simulink model "control_pra"  (R2021a)
settings: Solver=FixedStepDiscrete  StartTime=0.0  StopTime=10  FixedStep=0.005  RelTol=1e-3  EnableMultiTasking=on
PreLoadFcn:
  | disp(pwd)
PostLoadFcn:
  | c2000demoscallback(1)
undefined symbols (not defined in the file): CommandConstEnable, CommandData, FrameData, MailBoxRx, MailBoxTx, SCIAReceivedComplete, StatusConstClose, StatusConstClosed, StatusConstError, StatusConstHoming, StatusConstIdle, StatusConstPaused, StatusConstReady, StatusConstReset, StatusConstRunning, StatusConstStart, StatusConstStopped, StatusData
libraries: simulink x30, c280xlib x19, idelinklib_common x16, c2000lib x1, c2833xlib x1
(part 3 of 3)

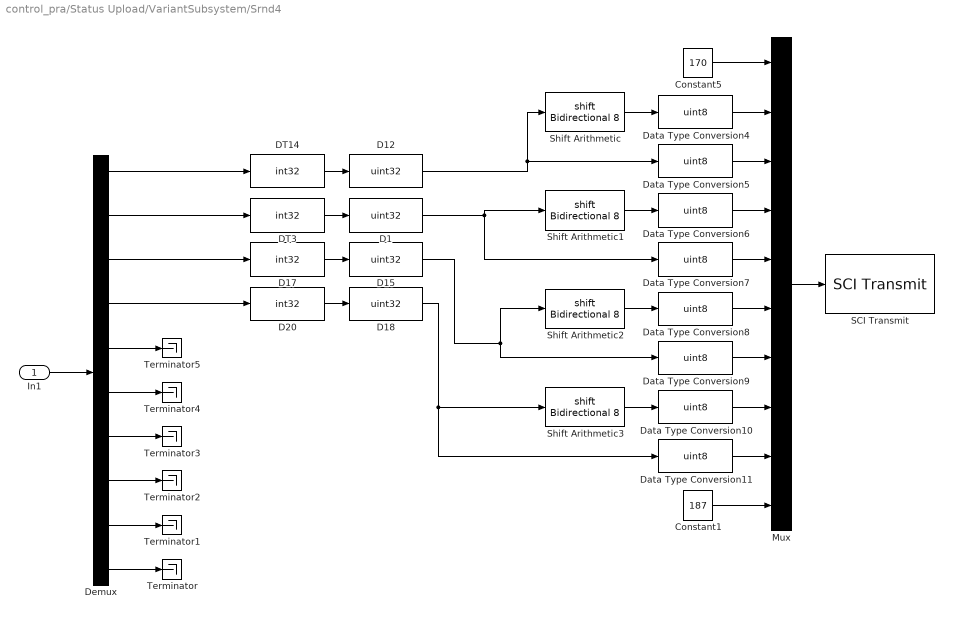
== system control_pra/Status Upload/VariantSubsystem/Srnd4 ==
  In1 : Inport
  Constant1 : Constant  Value=187  OutDataTypeStr=uint8
  Constant5 : Constant  Value=170  OutDataTypeStr=uint8
  D{1,12,15,18} (4 alike) : DataTypeConversion  OutDataTypeStr=uint32
  D17 : DataTypeConversion  OutDataTypeStr=int32
  D20 : DataTypeConversion  OutDataTypeStr=int32
  DT14 : DataTypeConversion  OutDataTypeStr=int32
  DT3 : DataTypeConversion  OutDataTypeStr=int32
  Data Type Conversion{4..11} (8 alike) : DataTypeConversion  OutDataTypeStr=uint8
  Demux : Demux  Outputs=10
  Mux : Mux  Inputs=10
  SCI Transmit : c280xlib/SCI Transmit  sciModule=A  dataHead=''  dataTail=''  postInterrupt=on  numFifo=16
  Shift Arithmetic{,1..3} (4 alike) : ArithShift  BitShiftNumber=8
  Terminator{,1..5} (6 alike) : Terminator
  wires:
  In1/1 -> Demux/1
  Demux/3 -> D17/1
  Demux/1 -> DT14/1
  Demux/2 -> DT3/1
  Demux/4 -> D20/1
  Demux/10 -> Terminator/1
  Demux/9 -> Terminator1/1
  Demux/8 -> Terminator2/1
  Demux/7 -> Terminator3/1
  Demux/6 -> Terminator4/1
  Demux/5 -> Terminator5/1
  DT14/1 -> D12/1
  DT3/1 -> D1/1
  D17/1 -> D15/1
  D20/1 -> D18/1
  Data Type Conversion11/1 -> Mux/9
  Data Type Conversion9/1 -> Mux/7
  Shift Arithmetic2/1 -> Data Type Conversion8/1
  Data Type Conversion7/1 -> Mux/5
  D18/1 -> Data Type Conversion11/1, Shift Arithmetic3/1
  D1/1 -> Data Type Conversion7/1, Shift Arithmetic1/1
  Shift Arithmetic/1 -> Data Type Conversion4/1
  Data Type Conversion8/1 -> Mux/6
  Constant1/1 -> Mux/10
  Data Type Conversion4/1 -> Mux/2
  Shift Arithmetic3/1 -> Data Type Conversion10/1
  Data Type Conversion6/1 -> Mux/4
  Constant5/1 -> Mux/1
  Mux/1 -> SCI Transmit/1
  D15/1 -> Data Type Conversion9/1, Shift Arithmetic2/1
  D12/1 -> Shift Arithmetic/1, Data Type Conversion5/1
  Data Type Conversion5/1 -> Mux/3
  Data Type Conversion10/1 -> Mux/8
  Shift Arithmetic1/1 -> Data Type Conversion6/1

== system control_pra/System Config/CAN_Config_C/Model Header ==

== system control_pra/System Config/CAN_Config_C/Model Source1 ==

== system control_pra/System Config/CAN_Config_C/System Initialize1 ==

== system control_pra/System Config/CAN_Config_S/Model Header ==

== system control_pra/System Config/CAN_Config_S/Model Source1 ==

== system control_pra/System Config/CAN_Config_S/Subsystem ==
  Enable : EnablePort
  eCANAM0 : c280xlib/eCAN Transmit  chipFamily=C280x  useModule=eCAN_A  mailboxNo=0  messageID=hex2dec('300')  messageType=Standard (11-bit identifier)  enableBlockingMode=off  postInterrupt=off  interruptLine=0
      settings: SourceProductBaseCode=TIC2000
  eCANAM1 : c280xlib/eCAN Transmit  chipFamily=C280x  useModule=eCAN_A  mailboxNo=1  messageID=hex2dec('301')  messageType=Standard (11-bit identifier)  enableBlockingMode=off  postInterrupt=off  interruptLine=0
      settings: SourceProductBaseCode=TIC2000
  eCANAM2 : c280xlib/eCAN Transmit  Commented=on  chipFamily=C280x  useModule=eCAN_A  mailboxNo=2  messageID=hex2dec('301')  messageType=Standard (11-bit identifier)  enableBlockingMode=off  postInterrupt=off  interruptLine=0
      settings: SourceProductBaseCode=TIC2000
  eCANAM3 : c280xlib/eCAN Transmit  Commented=on  chipFamily=C280x  useModule=eCAN_A  mailboxNo=3  messageID=hex2dec('303')  messageType=Standard (11-bit identifier)  enableBlockingMode=off  postInterrupt=off  interruptLine=0
      settings: SourceProductBaseCode=TIC2000
  eCANAM4 : c280xlib/eCAN Receive  chipFamily=C280x  useModule=eCAN_A  mailboxNo=4  messageID=hex2dec('281')  messageType=Standard (11-bit identifier)  sampleTime=-1  dataType=uint16  initValue=0  outputMessageLength=off  outputMessageTimeStamp=off  postInterrupt=off  interruptLine=0
      settings: SourceProductBaseCode=TIC2000
  eCANAM5 : c280xlib/eCAN Receive  Commented=on  chipFamily=C280x  useModule=eCAN_A  mailboxNo=5  messageID=hex2dec('281')  messageType=Standard (11-bit identifier)  sampleTime=-1  dataType=uint16  initValue=0  outputMessageLength=off  outputMessageTimeStamp=off  postInterrupt=off  interruptLine=0
      settings: SourceProductBaseCode=TIC2000
  eCANAM6 : c280xlib/eCAN Receive  Commented=on  chipFamily=C280x  useModule=eCAN_A  mailboxNo=6  messageID=hex2dec('283')  messageType=Standard (11-bit identifier)  sampleTime=-1  dataType=uint16  initValue=0  outputMessageLength=off  outputMessageTimeStamp=off  postInterrupt=off  interruptLine=0
      settings: SourceProductBaseCode=TIC2000
  eCANBM0 : c280xlib/eCAN Transmit  Commented=on  chipFamily=C280x  useModule=eCAN_B  mailboxNo=0  messageID=hex2dec('300')  messageType=Standard (11-bit identifier)  enableBlockingMode=off  postInterrupt=off  interruptLine=0
      settings: SourceProductBaseCode=TIC2000
  eCANBM1 : c280xlib/eCAN Transmit  Commented=on  chipFamily=C280x  useModule=eCAN_B  mailboxNo=1  messageID=hex2dec('304')  messageType=Standard (11-bit identifier)  enableBlockingMode=off  postInterrupt=off  interruptLine=0
      settings: SourceProductBaseCode=TIC2000
  eCANBM2 : c280xlib/eCAN Transmit  Commented=on  chipFamily=C280x  useModule=eCAN_B  mailboxNo=2  messageID=hex2dec('305')  messageType=Standard (11-bit identifier)  enableBlockingMode=off  postInterrupt=off  interruptLine=0
      settings: SourceProductBaseCode=TIC2000
  eCANBM3 : c280xlib/eCAN Transmit  Commented=on  chipFamily=C280x  useModule=eCAN_B  mailboxNo=3  messageID=hex2dec('306')  messageType=Standard (11-bit identifier)  enableBlockingMode=off  postInterrupt=off  interruptLine=0
      settings: SourceProductBaseCode=TIC2000
  eCANBM4 : c280xlib/eCAN Receive  Commented=on  chipFamily=C280x  useModule=eCAN_B  mailboxNo=4  messageID=hex2dec('284')  messageType=Standard (11-bit identifier)  sampleTime=-1  dataType=uint16  initValue=0  outputMessageLength=off  outputMessageTimeStamp=off  postInterrupt=off  interruptLine=0
      settings: SourceProductBaseCode=TIC2000
  eCANBM5 : c280xlib/eCAN Receive  Commented=on  chipFamily=C280x  useModule=eCAN_B  mailboxNo=5  messageID=hex2dec('285')  messageType=Standard (11-bit identifier)  sampleTime=-1  dataType=uint16  initValue=0  outputMessageLength=off  outputMessageTimeStamp=off  postInterrupt=off  interruptLine=0
      settings: SourceProductBaseCode=TIC2000
  eCANBM6 : c280xlib/eCAN Receive  Commented=on  chipFamily=C280x  useModule=eCAN_B  mailboxNo=6  messageID=hex2dec('286')  messageType=Standard (11-bit identifier)  sampleTime=-1  dataType=uint16  initValue=0  outputMessageLength=off  outputMessageTimeStamp=off  postInterrupt=off  interruptLine=0
      settings: SourceProductBaseCode=TIC2000

== system control_pra/System Config/CAN_Config_S/System Initialize1 ==

== system control_pra/System Config/CAN_Config_S/eCANA Transmit1 ==
  Data : Inport
  Constant1 : Constant  Value=MailBox  OutDataTypeStr=uint8  SampleTime=-1
  Memory Copy : idelinklib_common/Memory Copy  copyFrom=Input port  copyFromAddressSource=Specify via dialog  copyFromAddress=hex2dec('00001000')  copyFromSrcCode=myVariableSrc  dataTypeFrom=Inherit from input port  dataDimensionFrom=4  useOffsetFrom=off  offsetFromSrc=Specify via dialog  offsetFrom=0  strideFrom=1  copyTo=Specified source code symbol  copyToAddressSource=Specify via dialog  copyToAddress=hex2dec('00002000')  copyToSrcCode=&CanAMsg.TxWord  dataTypeTo=uint16  useOffsetTo=off  offsetToSrc=Specify via dialog  offsetTo=0  strideTo=1  sampleTime=-1  useInitValue=off  initValueSrc=Specify constant value  initValue=1  initValueSrcCode=myInitValueVariable  useAsMask=off  maskOperator=bitwise AND  useTermValue=off  termValue=1  isRealtimeEnabled=off  emitCCBeforeWrite=off  CCBeforeWrite=/* Custom Code Before Write*/  emitCCAfterWrite=off  CCAfterWrite=/* Custom Code After Write*/  useDMACopy=off  enableBlockingMode=off
      settings: SourceProductBaseCode=ME
  Memory Copy1 : idelinklib_common/Memory Copy  copyFrom=Input port  copyFromAddressSource=Specify via dialog  copyFromAddress=hex2dec('00001000')  copyFromSrcCode=myVariableSrc  dataTypeFrom=Inherit from input port  dataDimensionFrom=1  useOffsetFrom=off  offsetFromSrc=Specify via dialog  offsetFrom=0  strideFrom=1  copyTo=Specified source code symbol  copyToAddressSource=Specify via dialog  copyToAddress=hex2dec('00002000')  copyToSrcCode=&CanAMsg.MailBox  dataTypeTo=uint8  useOffsetTo=off  offsetToSrc=Specify via dialog  offsetTo=0  strideTo=1  sampleTime=-1  useInitValue=off  initValueSrc=Specify constant value  initValue=1  initValueSrcCode=myInitValueVariable  useAsMask=off  maskOperator=bitwise AND  useTermValue=off  termValue=1  isRealtimeEnabled=off  emitCCBeforeWrite=off  CCBeforeWrite=/* Custom Code Before Write*/  emitCCAfterWrite=off  CCAfterWrite=/* Custom Code After Write*/  useDMACopy=off  enableBlockingMode=off
      settings: SourceProductBaseCode=ME
  System Outputs : Subsystem  mask(System Outputs){MailBox=0}
      settings: CopyFcn=cccopyfcn(gcb)  OpenFcn=ccopenfcn('System Outputs Function')
      mask Help: eval('feval(''rtwprivate'',''rtwhelpview'',''rtw_sys_outputs_block'')');
      mask TypeOptions MailBox: 0 | 1 | 2 | 3 | 4 | 5
  wires:
  Data/1 -> Memory Copy/1
  Constant1/1 -> Memory Copy1/1

== system control_pra/System Config/CAN_Config_S/eCANA Transmit2 ==
  Data : Inport
  Constant1 : Constant  Value=MailBox  OutDataTypeStr=uint8  SampleTime=-1
  Memory Copy : idelinklib_common/Memory Copy  copyFrom=Input port  copyFromAddressSource=Specify via dialog  copyFromAddress=hex2dec('00001000')  copyFromSrcCode=myVariableSrc  dataTypeFrom=Inherit from input port  dataDimensionFrom=4  useOffsetFrom=off  offsetFromSrc=Specify via dialog  offsetFrom=0  strideFrom=1  copyTo=Specified source code symbol  copyToAddressSource=Specify via dialog  copyToAddress=hex2dec('00002000')  copyToSrcCode=&CanAMsg.TxWord  dataTypeTo=uint16  useOffsetTo=off  offsetToSrc=Specify via dialog  offsetTo=0  strideTo=1  sampleTime=-1  useInitValue=off  initValueSrc=Specify constant value  initValue=1  initValueSrcCode=myInitValueVariable  useAsMask=off  maskOperator=bitwise AND  useTermValue=off  termValue=1  isRealtimeEnabled=off  emitCCBeforeWrite=off  CCBeforeWrite=/* Custom Code Before Write*/  emitCCAfterWrite=off  CCAfterWrite=/* Custom Code After Write*/  useDMACopy=off  enableBlockingMode=off
      settings: SourceProductBaseCode=ME
  Memory Copy1 : idelinklib_common/Memory Copy  copyFrom=Input port  copyFromAddressSource=Specify via dialog  copyFromAddress=hex2dec('00001000')  copyFromSrcCode=myVariableSrc  dataTypeFrom=Inherit from input port  dataDimensionFrom=1  useOffsetFrom=off  offsetFromSrc=Specify via dialog  offsetFrom=0  strideFrom=1  copyTo=Specified source code symbol  copyToAddressSource=Specify via dialog  copyToAddress=hex2dec('00002000')  copyToSrcCode=&CanAMsg.MailBox  dataTypeTo=uint8  useOffsetTo=off  offsetToSrc=Specify via dialog  offsetTo=0  strideTo=1  sampleTime=-1  useInitValue=off  initValueSrc=Specify constant value  initValue=1  initValueSrcCode=myInitValueVariable  useAsMask=off  maskOperator=bitwise AND  useTermValue=off  termValue=1  isRealtimeEnabled=off  emitCCBeforeWrite=off  CCBeforeWrite=/* Custom Code Before Write*/  emitCCAfterWrite=off  CCAfterWrite=/* Custom Code After Write*/  useDMACopy=off  enableBlockingMode=off
      settings: SourceProductBaseCode=ME
  System Outputs : Subsystem  mask(System Outputs){MailBox=0}
      settings: CopyFcn=cccopyfcn(gcb)  OpenFcn=ccopenfcn('System Outputs Function')
      mask Help: eval('feval(''rtwprivate'',''rtwhelpview'',''rtw_sys_outputs_block'')');
      mask TypeOptions MailBox: 0 | 1 | 2 | 3 | 4 | 5
  wires:
  Constant1/1 -> Memory Copy1/1
  Data/1 -> Memory Copy/1

== system control_pra/System Config/CAN_Config_S/eCANA Transmit3 ==
  Data : Inport
  Constant1 : Constant  Value=MailBox  OutDataTypeStr=uint8  SampleTime=-1
  Memory Copy : idelinklib_common/Memory Copy  copyFrom=Input port  copyFromAddressSource=Specify via dialog  copyFromAddress=hex2dec('00001000')  copyFromSrcCode=myVariableSrc  dataTypeFrom=Inherit from input port  dataDimensionFrom=4  useOffsetFrom=off  offsetFromSrc=Specify via dialog  offsetFrom=0  strideFrom=1  copyTo=Specified source code symbol  copyToAddressSource=Specify via dialog  copyToAddress=hex2dec('00002000')  copyToSrcCode=&CanAMsg.TxWord  dataTypeTo=uint16  useOffsetTo=off  offsetToSrc=Specify via dialog  offsetTo=0  strideTo=1  sampleTime=-1  useInitValue=off  initValueSrc=Specify constant value  initValue=1  initValueSrcCode=myInitValueVariable  useAsMask=off  maskOperator=bitwise AND  useTermValue=off  termValue=1  isRealtimeEnabled=off  emitCCBeforeWrite=off  CCBeforeWrite=/* Custom Code Before Write*/  emitCCAfterWrite=off  CCAfterWrite=/* Custom Code After Write*/  useDMACopy=off  enableBlockingMode=off
      settings: SourceProductBaseCode=ME
  Memory Copy1 : idelinklib_common/Memory Copy  copyFrom=Input port  copyFromAddressSource=Specify via dialog  copyFromAddress=hex2dec('00001000')  copyFromSrcCode=myVariableSrc  dataTypeFrom=Inherit from input port  dataDimensionFrom=1  useOffsetFrom=off  offsetFromSrc=Specify via dialog  offsetFrom=0  strideFrom=1  copyTo=Specified source code symbol  copyToAddressSource=Specify via dialog  copyToAddress=hex2dec('00002000')  copyToSrcCode=&CanAMsg.MailBox  dataTypeTo=uint8  useOffsetTo=off  offsetToSrc=Specify via dialog  offsetTo=0  strideTo=1  sampleTime=-1  useInitValue=off  initValueSrc=Specify constant value  initValue=1  initValueSrcCode=myInitValueVariable  useAsMask=off  maskOperator=bitwise AND  useTermValue=off  termValue=1  isRealtimeEnabled=off  emitCCBeforeWrite=off  CCBeforeWrite=/* Custom Code Before Write*/  emitCCAfterWrite=off  CCAfterWrite=/* Custom Code After Write*/  useDMACopy=off  enableBlockingMode=off
      settings: SourceProductBaseCode=ME
  System Outputs : Subsystem  mask(System Outputs){MailBox=0}
      settings: CopyFcn=cccopyfcn(gcb)  OpenFcn=ccopenfcn('System Outputs Function')
      mask Help: eval('feval(''rtwprivate'',''rtwhelpview'',''rtw_sys_outputs_block'')');
      mask TypeOptions MailBox: 0 | 1 | 2 | 3 | 4 | 5
  wires:
  Data/1 -> Memory Copy/1
  Constant1/1 -> Memory Copy1/1

== system control_pra/System Config/CAN_Config_S/eCANB Transmit1 ==
  Data : Inport
  Constant1 : Constant  Value=MailBox  OutDataTypeStr=uint8  SampleTime=-1
  Memory Copy : idelinklib_common/Memory Copy  copyFrom=Input port  copyFromAddressSource=Specify via dialog  copyFromAddress=hex2dec('00001000')  copyFromSrcCode=myVariableSrc  dataTypeFrom=Inherit from input port  dataDimensionFrom=4  useOffsetFrom=off  offsetFromSrc=Specify via dialog  offsetFrom=0  strideFrom=1  copyTo=Specified source code symbol  copyToAddressSource=Specify via dialog  copyToAddress=hex2dec('00002000')  copyToSrcCode=&CanBMsg.TxWord  dataTypeTo=uint16  useOffsetTo=off  offsetToSrc=Specify via dialog  offsetTo=0  strideTo=1  sampleTime=-1  useInitValue=off  initValueSrc=Specify constant value  initValue=1  initValueSrcCode=myInitValueVariable  useAsMask=off  maskOperator=bitwise AND  useTermValue=off  termValue=1  isRealtimeEnabled=off  emitCCBeforeWrite=off  CCBeforeWrite=/* Custom Code Before Write*/  emitCCAfterWrite=off  CCAfterWrite=/* Custom Code After Write*/  useDMACopy=off  enableBlockingMode=off
      settings: SourceProductBaseCode=ME
  Memory Copy1 : idelinklib_common/Memory Copy  copyFrom=Input port  copyFromAddressSource=Specify via dialog  copyFromAddress=hex2dec('00001000')  copyFromSrcCode=myVariableSrc  dataTypeFrom=Inherit from input port  dataDimensionFrom=1  useOffsetFrom=off  offsetFromSrc=Specify via dialog  offsetFrom=0  strideFrom=1  copyTo=Specified source code symbol  copyToAddressSource=Specify via dialog  copyToAddress=hex2dec('00002000')  copyToSrcCode=&CanBMsg.MailBox  dataTypeTo=uint8  useOffsetTo=off  offsetToSrc=Specify via dialog  offsetTo=0  strideTo=1  sampleTime=-1  useInitValue=off  initValueSrc=Specify constant value  initValue=1  initValueSrcCode=myInitValueVariable  useAsMask=off  maskOperator=bitwise AND  useTermValue=off  termValue=1  isRealtimeEnabled=off  emitCCBeforeWrite=off  CCBeforeWrite=/* Custom Code Before Write*/  emitCCAfterWrite=off  CCAfterWrite=/* Custom Code After Write*/  useDMACopy=off  enableBlockingMode=off
      settings: SourceProductBaseCode=ME
  System Outputs : Subsystem  mask(System Outputs){ShowInLibBrowser=0}
      mask prompts: ShowInLibBrowser "Simulink:masks:CustCodeMaskParam1_MP"
      settings: CopyFcn=cccopyfcn(gcb)  OpenFcn=ccopenfcn('System Outputs Function')
      mask Help: eval('feval(''rtwprivate'',''rtwhelpview'',''rtw_sys_outputs_block'')');
      mask DialogControl ShowInLibBrowser Prompt: Mask Parameter 1:
      mask Display: disp('System\nOutputs');
  wires:
  Constant1/1 -> Memory Copy1/1
  Data/1 -> Memory Copy/1

== system control_pra/System Config/CAN_Config_S/eCANB Transmit2 ==
  Data : Inport
  Constant1 : Constant  Value=MailBox  OutDataTypeStr=uint8  SampleTime=-1
  Memory Copy : idelinklib_common/Memory Copy  copyFrom=Input port  copyFromAddressSource=Specify via dialog  copyFromAddress=hex2dec('00001000')  copyFromSrcCode=myVariableSrc  dataTypeFrom=Inherit from input port  dataDimensionFrom=4  useOffsetFrom=off  offsetFromSrc=Specify via dialog  offsetFrom=0  strideFrom=1  copyTo=Specified source code symbol  copyToAddressSource=Specify via dialog  copyToAddress=hex2dec('00002000')  copyToSrcCode=&CanBMsg.TxWord  dataTypeTo=uint16  useOffsetTo=off  offsetToSrc=Specify via dialog  offsetTo=0  strideTo=1  sampleTime=-1  useInitValue=off  initValueSrc=Specify constant value  initValue=1  initValueSrcCode=myInitValueVariable  useAsMask=off  maskOperator=bitwise AND  useTermValue=off  termValue=1  isRealtimeEnabled=off  emitCCBeforeWrite=off  CCBeforeWrite=/* Custom Code Before Write*/  emitCCAfterWrite=off  CCAfterWrite=/* Custom Code After Write*/  useDMACopy=off  enableBlockingMode=off
      settings: SourceProductBaseCode=ME
  Memory Copy1 : idelinklib_common/Memory Copy  copyFrom=Input port  copyFromAddressSource=Specify via dialog  copyFromAddress=hex2dec('00001000')  copyFromSrcCode=myVariableSrc  dataTypeFrom=Inherit from input port  dataDimensionFrom=1  useOffsetFrom=off  offsetFromSrc=Specify via dialog  offsetFrom=0  strideFrom=1  copyTo=Specified source code symbol  copyToAddressSource=Specify via dialog  copyToAddress=hex2dec('00002000')  copyToSrcCode=&CanBMsg.MailBox  dataTypeTo=uint8  useOffsetTo=off  offsetToSrc=Specify via dialog  offsetTo=0  strideTo=1  sampleTime=-1  useInitValue=off  initValueSrc=Specify constant value  initValue=1  initValueSrcCode=myInitValueVariable  useAsMask=off  maskOperator=bitwise AND  useTermValue=off  termValue=1  isRealtimeEnabled=off  emitCCBeforeWrite=off  CCBeforeWrite=/* Custom Code Before Write*/  emitCCAfterWrite=off  CCAfterWrite=/* Custom Code After Write*/  useDMACopy=off  enableBlockingMode=off
      settings: SourceProductBaseCode=ME
  System Outputs : Subsystem  mask(System Outputs){ShowInLibBrowser=0}
      mask prompts: ShowInLibBrowser "Simulink:masks:CustCodeMaskParam1_MP"
      settings: CopyFcn=cccopyfcn(gcb)  OpenFcn=ccopenfcn('System Outputs Function')
      mask Help: eval('feval(''rtwprivate'',''rtwhelpview'',''rtw_sys_outputs_block'')');
      mask DialogControl ShowInLibBrowser Prompt: Mask Parameter 1:
      mask Display: disp('System\nOutputs');
  wires:
  Data/1 -> Memory Copy/1
  Constant1/1 -> Memory Copy1/1

== system control_pra/System Config/CAN_Config_S/eCANB Transmit3 ==
  Data : Inport
  Constant1 : Constant  Value=MailBox  OutDataTypeStr=uint8  SampleTime=-1
  Memory Copy : idelinklib_common/Memory Copy  copyFrom=Input port  copyFromAddressSource=Specify via dialog  copyFromAddress=hex2dec('00001000')  copyFromSrcCode=myVariableSrc  dataTypeFrom=Inherit from input port  dataDimensionFrom=4  useOffsetFrom=off  offsetFromSrc=Specify via dialog  offsetFrom=0  strideFrom=1  copyTo=Specified source code symbol  copyToAddressSource=Specify via dialog  copyToAddress=hex2dec('00002000')  copyToSrcCode=&CanBMsg.TxWord  dataTypeTo=uint16  useOffsetTo=off  offsetToSrc=Specify via dialog  offsetTo=0  strideTo=1  sampleTime=-1  useInitValue=off  initValueSrc=Specify constant value  initValue=1  initValueSrcCode=myInitValueVariable  useAsMask=off  maskOperator=bitwise AND  useTermValue=off  termValue=1  isRealtimeEnabled=off  emitCCBeforeWrite=off  CCBeforeWrite=/* Custom Code Before Write*/  emitCCAfterWrite=off  CCAfterWrite=/* Custom Code After Write*/  useDMACopy=off  enableBlockingMode=off
      settings: SourceProductBaseCode=ME
  Memory Copy1 : idelinklib_common/Memory Copy  copyFrom=Input port  copyFromAddressSource=Specify via dialog  copyFromAddress=hex2dec('00001000')  copyFromSrcCode=myVariableSrc  dataTypeFrom=Inherit from input port  dataDimensionFrom=1  useOffsetFrom=off  offsetFromSrc=Specify via dialog  offsetFrom=0  strideFrom=1  copyTo=Specified source code symbol  copyToAddressSource=Specify via dialog  copyToAddress=hex2dec('00002000')  copyToSrcCode=&CanBMsg.MailBox  dataTypeTo=uint8  useOffsetTo=off  offsetToSrc=Specify via dialog  offsetTo=0  strideTo=1  sampleTime=-1  useInitValue=off  initValueSrc=Specify constant value  initValue=1  initValueSrcCode=myInitValueVariable  useAsMask=off  maskOperator=bitwise AND  useTermValue=off  termValue=1  isRealtimeEnabled=off  emitCCBeforeWrite=off  CCBeforeWrite=/* Custom Code Before Write*/  emitCCAfterWrite=off  CCAfterWrite=/* Custom Code After Write*/  useDMACopy=off  enableBlockingMode=off
      settings: SourceProductBaseCode=ME
  System Outputs : Subsystem  mask(System Outputs){ShowInLibBrowser=0}
      mask prompts: ShowInLibBrowser "Simulink:masks:CustCodeMaskParam1_MP"
      settings: CopyFcn=cccopyfcn(gcb)  OpenFcn=ccopenfcn('System Outputs Function')
      mask Help: eval('feval(''rtwprivate'',''rtwhelpview'',''rtw_sys_outputs_block'')');
      mask DialogControl ShowInLibBrowser Prompt: Mask Parameter 1:
      mask Display: disp('System\nOutputs');
  wires:
  Constant1/1 -> Memory Copy1/1
  Data/1 -> Memory Copy/1

== system control_pra/System Config/HC595_Config/Model Header ==

== system control_pra/System Config/HC595_Config/Model Source ==

== system control_pra/System Config/HC595_Config/System Initialize1 ==

== system control_pra/System Config/LCD_Config/Model Header ==

== system control_pra/System Config/LCD_Config/Model Source ==

== system control_pra/System Config/LCD_Config/System Initialize ==

== system control_pra/System Config/SCI_Config/Model Header ==

== system control_pra/System Config/SCI_Config/Model Source ==

== system control_pra/Command Download/SCIA_RX_Process/Process/Enabled Subsystem ==
  Enable : EnablePort
  Data Store Read1 : DataStoreRead  DataStoreName=FrameData  DataStoreElements=FrameData(2:17)  IndexOptions=Index vector (dialog)  Indices=1  OutputSizes=1
  Data Store Read2 : DataStoreRead  DataStoreName=FrameData  DataStoreElements=FrameData(1)  IndexOptions=Index vector (dialog)  Indices=1  OutputSizes=1
  Data Store Write : DataStoreWrite  DataStoreName=Command  IndexOptions=Index vector (dialog)  Indices=1  OutputSizes=1
  Data Store Write1 : DataStoreWrite  DataStoreName=CommandData  IndexOptions=Index vector (dialog)  Indices=1  OutputSizes=1
  Data Type Conversion : DataTypeConversion  OutDataTypeStr=double
  PositionIntToFloat : Subsystem  TreatAsAtomicUnit=on
  wires:
  Data Store Read2/1 -> Data Store Write/1
  Data Store Read1/1 -> PositionIntToFloat/1(Data)
  PositionIntToFloat/1(Out1) -> Data Type Conversion/1
  Data Type Conversion/1 -> Data Store Write1/1

== system control_pra/Command Download/SCIA_RX_Process/Process/System Outputs ==

== system control_pra/MotionControl/Reset/AI=0/eCANA Transmit/System Outputs ==

== system control_pra/MotionControl/Reset/AI=1/eCANA Receive/System Outputs ==

== system control_pra/MotionControl/Reset/AI=1/eCANA Transmit/System Outputs ==

== system control_pra/MotionControl/Reset/BG /eCANA Transmit/System Outputs ==

== system control_pra/MotionControl/Reset/JV=0/eCANA Transmit/System Outputs ==

== system control_pra/MotionControl/Reset/MO=0/eCANA Transmit/System Outputs ==

== system control_pra/MotionControl/Reset/MO=1/eCANA Transmit/System Outputs ==

== system control_pra/MotionControl/Reset/PX/eCANA Transmit/System Outputs ==

== system control_pra/MotionControl/Reset/Set_P0/eCANA Receive/System Outputs ==

== system control_pra/MotionControl/Reset/UM=4/eCANA Transmit/System Outputs ==

== system control_pra/MotionControl/Start/BG/eCANA Transmit/System Outputs ==

== system control_pra/MotionControl/Start/MO=1/eCANA Transmit/System Outputs ==

== system control_pra/MotionControl/Start/UM=1or4/eCANA Transmit/System Outputs ==

== system control_pra/Pendulum/Subsystem/CanReceive/Subsystem1 ==
  Current : Inport
  PosL : Inport  Port=2
  PosH : Inport  Port=3
  Enable : EnablePort
  Add : Sum
  Data Store Write : DataStoreWrite  DataStoreName=Motor_Current  IndexOptions=Index vector (dialog)  Indices=1  OutputSizes=1
  Data Store Write1 : DataStoreWrite  DataStoreName=Motor_Position  IndexOptions=Index vector (dialog)  Indices=1  OutputSizes=1
  Data Type Conversion : DataTypeConversion  OutDataTypeStr=int32
  Data Type Conversion2 : DataTypeConversion  OutDataTypeStr=int32
  Gain2 : Gain  Gain=0.001  OutDataTypeStr=double
  Shift Arithmetic1 : ArithShift  BitShiftNumber=16  BitShiftDirection=Left
  wires:
  Data Type Conversion/1 -> Add/1
  Data Type Conversion2/1 -> Shift Arithmetic1/1
  Add/1 -> Gain2/1
  Shift Arithmetic1/1 -> Add/2
  Current/1 -> Data Store Write/1
  PosL/1 -> Data Type Conversion/1
  PosH/1 -> Data Type Conversion2/1
  Gain2/1 -> Data Store Write1/1

== system control_pra/Pendulum/Subsystem/eCANA Receive/System Outputs ==

== system control_pra/Pendulum/Subsystem/eCANA Transmit/System Outputs ==

== system control_pra/Status Display/Enabled Subsystem/Status Display/System Outputs ==

== system control_pra/Status Display/Enabled Subsystem/Status Display/数码显示 ==
  SEG1 : Inport  OutDataTypeStr=uint8
  SEG2 : Inport  Port=2  OutDataTypeStr=uint8
  SEG3 : Inport  Port=3  OutDataTypeStr=uint8
  SEG4 : Inport  Port=4  OutDataTypeStr=uint8
  Memory Copy1 : idelinklib_common/Memory Copy  copyFrom=Input port  copyFromAddressSource=Specify via dialog  copyFromAddress=hex2dec('00001000')  copyFromSrcCode=myVariableSrc  dataTypeFrom=uint8  dataDimensionFrom=4  useOffsetFrom=off  offsetFromSrc=Specify via dialog  offsetFrom=0  strideFrom=1  copyTo=Specified source code symbol  copyToAddressSource=Specify via dialog  copyToAddress=hex2dec('00002000')  copyToSrcCode=SEG  dataTypeTo=uint8  useOffsetTo=off  offsetToSrc=Specify via dialog  offsetTo=0  strideTo=1  sampleTime=-1  useInitValue=off  initValueSrc=Specify constant value  initValue=1  initValueSrcCode=myInitValueVariable  useAsMask=off  maskOperator=bitwise AND  useTermValue=off  termValue=1  isRealtimeEnabled=off  emitCCBeforeWrite=off  CCBeforeWrite=/* Custom Code Before Write*/  emitCCAfterWrite=off  CCAfterWrite=/* Custom Code After Write*/  useDMACopy=off  enableBlockingMode=off
      settings: SourceProductBaseCode=ME
  Mux : Mux
  System Outputs : Subsystem  mask(System Outputs){ShowInLibBrowser=0}
      mask prompts: ShowInLibBrowser "Simulink:masks:CustCodeMaskParam1_MP"
      settings: CopyFcn=cccopyfcn(gcb)  OpenFcn=ccopenfcn('System Outputs Function')
      mask Help: eval('feval(''rtwprivate'',''rtwhelpview'',''rtw_sys_outputs_block'')');
      mask Display: disp('System\nOutputs');
  wires:
  SEG3/1 -> Mux/3
  Mux/1 -> Memory Copy1/1
  SEG1/1 -> Mux/1
  SEG2/1 -> Mux/2
  SEG4/1 -> Mux/4

== system control_pra/System Config/CAN_Config_S/eCANA Transmit1/System Outputs ==

== system control_pra/System Config/CAN_Config_S/eCANA Transmit2/System Outputs ==

== system control_pra/System Config/CAN_Config_S/eCANA Transmit3/System Outputs ==

== system control_pra/System Config/CAN_Config_S/eCANB Transmit1/System Outputs ==

== system control_pra/System Config/CAN_Config_S/eCANB Transmit2/System Outputs ==

== system control_pra/System Config/CAN_Config_S/eCANB Transmit3/System Outputs ==

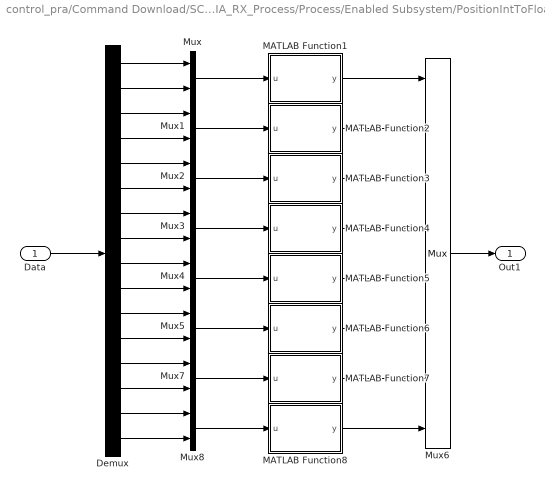
== system control_pra/Command Download/SCIA_RX_Process/Process/Enabled Subsystem/PositionIntToFloat ==
  Data : Inport
  Demux : Demux  Outputs=16
  MATLAB Function1 : MATLAB Function  TreatAsAtomicUnit=on
  MATLAB Function2 : MATLAB Function  TreatAsAtomicUnit=on
  MATLAB Function3 : MATLAB Function  TreatAsAtomicUnit=on
  MATLAB Function4 : MATLAB Function  TreatAsAtomicUnit=on
  MATLAB Function5 : MATLAB Function  TreatAsAtomicUnit=on
  MATLAB Function6 : MATLAB Function  TreatAsAtomicUnit=on
  MATLAB Function7 : MATLAB Function  TreatAsAtomicUnit=on
  MATLAB Function8 : MATLAB Function  TreatAsAtomicUnit=on
  Mux{,1..5,7..8} (8 alike) : Mux  Inputs=2
  Mux6 : Mux  Inputs=8
  Out1 : Outport
  wires:
  Demux/6 -> Mux2/2
  Demux/10 -> Mux4/2
  Mux5/1 -> MATLAB Function6/1(u)
  MATLAB Function6/1(y) -> Mux6/6
  MATLAB Function2/1(y) -> Mux6/2
  Mux2/1 -> MATLAB Function3/1(u)
  Demux/3 -> Mux1/1
  Data/1 -> Demux/1
  Demux/8 -> Mux3/2
  Demux/4 -> Mux1/2
  Mux3/1 -> MATLAB Function4/1(u)
  Demux/12 -> Mux5/2
  Mux1/1 -> MATLAB Function2/1(u)
  MATLAB Function3/1(y) -> Mux6/3
  Demux/11 -> Mux5/1
  Demux/7 -> Mux3/1
  MATLAB Function5/1(y) -> Mux6/5
  Demux/9 -> Mux4/1
  MATLAB Function4/1(y) -> Mux6/4
  Mux/1 -> MATLAB Function1/1(u)
  Demux/2 -> Mux/2
  Demux/5 -> Mux2/1
  MATLAB Function1/1(y) -> Mux6/1
  Demux/1 -> Mux/1
  Mux4/1 -> MATLAB Function5/1(u)
  Mux6/1 -> Out1/1
  MATLAB Function7/1(y) -> Mux6/7
  MATLAB Function8/1(y) -> Mux6/8
  Mux7/1 -> MATLAB Function7/1(u)
  Demux/13 -> Mux7/1
  Demux/14 -> Mux7/2
  Demux/15 -> Mux8/1
  Demux/16 -> Mux8/2
  Mux8/1 -> MATLAB Function8/1(u)

== system control_pra/Status Display/Enabled Subsystem/Status Display/数码显示/System Outputs ==

== matlab function control_pra/Status Upload/PositionFloatToInt/MATLAB Function7 ==
  data: u input; y output
function y = float2int(u)
y = zeros(1,2,'uint16');
y = typecast(single(u),'uint16');
end

== matlab function control_pra/Status Upload/PositionFloatToInt/MATLAB Function2 ==
  data: u input; y output
function y = float2int(u)
y = zeros(1,2,'uint16');
y = typecast(single(u),'uint16');
end

== matlab function control_pra/Status Upload/PositionFloatToInt/MATLAB Function1 ==
  data: u input; y output
function y = float2int(u)
y = zeros(1,2,'uint16');
y = typecast(single(u),'uint16');
end

== matlab function control_pra/Status Upload/PositionFloatToInt/MATLAB Function3 ==
  data: u input; y output
function y = float2int(u)
y = zeros(1,2,'uint16');
y = typecast(single(u),'uint16');
end

== matlab function control_pra/Status Upload/PositionFloatToInt/MATLAB Function4 ==
  data: u input; y output
function y = float2int(u)
y = zeros(1,2,'uint16');
y = typecast(single(u),'uint16');
end

== matlab function control_pra/Status Upload/PositionFloatToInt/MATLAB Function5 ==
  data: u input; y output
function y = float2int(u)
y = zeros(1,2,'uint16');
y = typecast(single(u),'uint16');
end

== matlab function control_pra/Status Upload/PositionFloatToInt/MATLAB Function6 ==
  data: u input; y output
function y = float2int(u)
y = zeros(1,2,'uint16');
y = typecast(single(u),'uint16');
end

== stateflow chart control_pra/MotionControl ==
  state CLOSED
    %关闭命令后-关闭状态
    entry:
    ControlStep=1;
    during:
    Status=Close()
    exit:
    ControlStep=0;
  state Initial [function]
  state STOPPED
    %停止运行后-停止状态
    entry:
    ControlStep=1;
    during:
    Status = Stop()
    exit:
    ControlStep=0;
  state INIT
    %上电后-初始化状态
    entry:
    Initial();
    exit:
  state Status = Idle [function]
  state Status = Reset [function]
  state RUNNING
    %开启运行后-运行状态
    entry:
    ControlStep=1;
    during:
    Status = Run()
    exit:
    ControlStep=0;
  state Status = Start [function]
  state STARTED
    %启动命令后-启动状态
    entry:
    ControlStep=1;
    during:
    Status=Start()
    exit:
    ControlStep=0;
  state READY
    %启动成功后-准备状态
    entry:
    ControlStep=1;
    during:
    Status=Ready()
    exit:
    ControlStep=0;
  state IDLE
    %初始化后-空闲状态
    entry:
    during:
    Status=Idle()
    exit:
  state Status = Ready [function]
  state Status = Home [function]
  state Status = Run [function]
  state RESET
    %复位命令后-复位状态
    entry:
    ControlStep=1;
    during:
    Status=Reset()
    exit:
    ControlStep=0;
  state HOMING
    %回零后-回零状态
    entry:
    ControlStep=1;
    during:
    Status=Home()
    exit:
    ControlStep=0;
  state Status = Stop [function]
  state ERROR
    %发生错误后-错误状态
    entry:
    during:
    exit:
  state Status = Close [function]
  (default) -> INIT
  READY -> CLOSED [order 3] : [Status==StatusConstClosed]
  CLOSED -> IDLE : [Status==StatusConstIdle]
  RUNNING -> STOPPED [order 2] : [Status==StatusConstStopped]
  STOPPED -> READY : [Status==StatusConstReady]
  INIT -> IDLE
  READY -> RUNNING [order 1] : [Status==StatusConstRunning]
  STARTED -> READY : [Status==StatusConstReady]
  IDLE -> STARTED [order 2] : [Status==StatusConstStart]
  ERROR -> READY : [Status==StatusConstReset]
  IDLE -> RESET [order 1] : [Status==StatusConstReset]
  RESET -> IDLE : [Status==StatusConstIdle]
  HOMING -> READY : [Status==StatusConstReady]
  READY -> HOMING [order 2] : [Status==StatusConstHoming]
  RUNNING -> ERROR [order 1] : [Status==StatusConstError]
  data: Status function_output uint16 size=[1 1]; Status function_output uint16 size=1; Status function_output uint16 size=1; Status function_output uint16 size=1; Status function_output uint16 size=1; Status function_output uint16 size=[1 1]; Status function_output uint16 size=[1 1]; Status function_output uint16 size=[1 1]; Status output uint16 size=[1 1] =uint16(0); ControlStep data_store_memory; StatusConstError parameter double; StatusConstReset parameter double; StatusConstRunning parameter double; StatusConstStart parameter double; StatusConstPaused parameter double; StatusConstIdle parameter double; StatusConstStopped parameter; StatusConstReady parameter; StatusConstHoming parameter; Command data_store_memory size=[1 1]; CommandData data_store_memory size=[1 8]; StatusConstClosed parameter

== matlab function control_pra/Command Download/SCIA_RX_Process/Process/Enabled Subsystem/PositionIntToFloat/MATLAB Function1 ==
  data: u input; y output
function y = int2float(u)
y = single(0);
y = typecast(u,'single');
end

== matlab function control_pra/Command Download/SCIA_RX_Process/Process/Enabled Subsystem/PositionIntToFloat/MATLAB Function2 ==
  data: u input; y output
function y = int2float(u)
y = single(0);
y = typecast(u,'single');
end

== matlab function control_pra/Command Download/SCIA_RX_Process/Process/Enabled Subsystem/PositionIntToFloat/MATLAB Function3 ==
  data: u input; y output
function y = int2float(u)
y = single(0);
y = typecast(u,'single');
end

== matlab function control_pra/Command Download/SCIA_RX_Process/Process/Enabled Subsystem/PositionIntToFloat/MATLAB Function4 ==
  data: u input; y output
function y = int2float(u)
y = single(0);
y = typecast(u,'single');
end

== matlab function control_pra/Command Download/SCIA_RX_Process/Process/Enabled Subsystem/PositionIntToFloat/MATLAB Function5 ==
  data: u input; y output
function y = int2float(u)
y = single(0);
y = typecast(u,'single');
end

== matlab function control_pra/Command Download/SCIA_RX_Process/Process/Enabled Subsystem/PositionIntToFloat/MATLAB Function6 ==
  data: u input; y output
function y = int2float(u)
y = single(0);
y = typecast(u,'single');
end

== matlab function control_pra/Command Download/SCIA_RX_Process/Process/Enabled Subsystem/PositionIntToFloat/MATLAB Function7 ==
  data: u input; y output
function y = int2float(u)
y = single(0);
y = typecast(u,'single');
end

== matlab function control_pra/Command Download/SCIA_RX_Process/Process/Enabled Subsystem/PositionIntToFloat/MATLAB Function8 ==
  data: u input; y output
function y = int2float(u)
y = single(0);
y = typecast(u,'single');
end

== matlab function control_pra/Status Upload/PositionFloatToInt/MATLAB Function8 ==
  data: u input; y output
function y = float2int(u)
y = zeros(1,2,'uint16');
y = typecast(single(u),'uint16');
end
